simulink model "Simple_wanderer_local"  (R2013a)
settings: Solver=FixedStepDiscrete  StartTime=0.0  StopTime=300000  FixedStep=0.1  RelTol=1e-3
StopFcn:
  | arrobot_stop
libraries: ariac x8, simulink x1
PauseFcn:
  | arrobot_stop
settings Model: Creator=reedh  LastModifiedBy=reedh
settings DataIOCC: SaveFormat=StructureWithTime

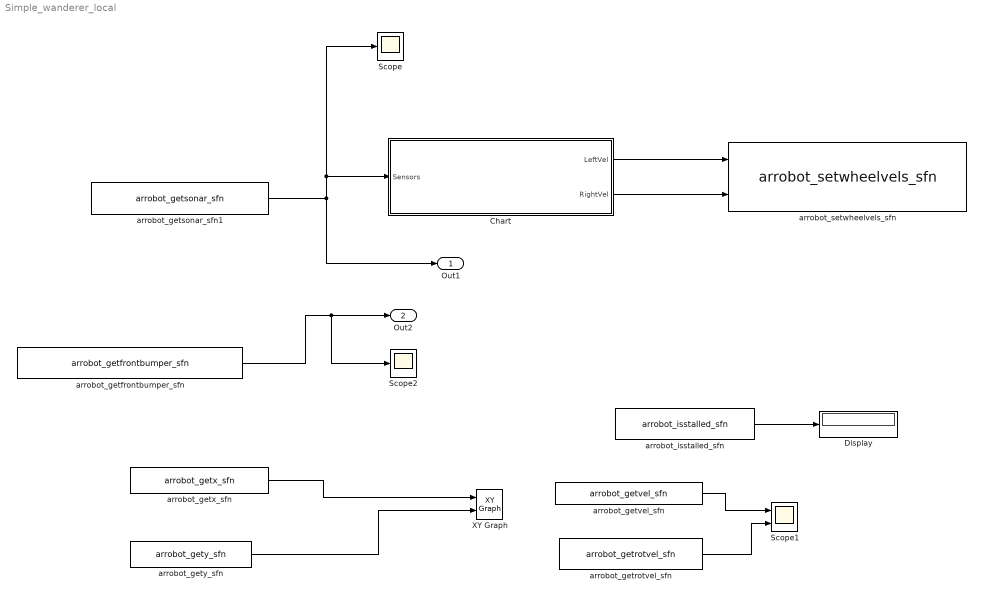
== system Simple_wanderer_local ==
  Chart : Stateflow chart  TreatAsAtomicUnit=on
  Display : Display
  Scope : Scope
      settings: YMin=0  YMax=5000
  Scope1 : Scope  NumInputPorts=2
      settings: YMin=-5~-5  YMax=5~5  SaveName=ScopeData2
  Scope2 : Scope
      settings: YMin=0  YMax=5000
  XY Graph : simulink/Sinks/XY Graph  xmin=-10000  xmax=10000  ymin=-10000  ymax=10000  st=100
  arrobot_getfrontbumper_sfn : ariac/arrobot_getfrontbumper_sfn  Description=Get range reading from one front bumper (0-indexed) of mobile robot  SFunctionSpec=int32 y1 = arrobot_get_front_bumper(int32 p1)  SParameter1=ones([1 1 ])  ShowSpec=on
      settings: AttributesFormatString=Get range reading from one front bumper (0-indexed) of mobile robot
  arrobot_getrotvel_sfn : ariac/arrobot_getrotvel_sfn  Description=Get current rotational velocity of mobile robot (deg/sec, counterclockwise +)  SFunctionSpec=double y1 = arrobot_getrotvel()  ShowSpec=on
      settings: AttributesFormatString=Get current rotational velocity of mobile robot (deg/sec, counterclockwise +)
  arrobot_getsonar_sfn1 : ariac/arrobot_getsonar_sfn  Description=Get range readings of all front sonar on mobile robot (mm)  SFunctionSpec=void arrobot_getsonar(double y1[16])  ShowSpec=on
      settings: AttributesFormatString=Get range readings of all front sonar on mobile robot (mm)
  arrobot_getvel_sfn : ariac/arrobot_getvel_sfn  Description=Get current forward/back velocity of mobile robot (mm/sec)  SFunctionSpec=double y1 = arrobot_getvel()  ShowSpec=on
      settings: AttributesFormatString=Get current forward/back velocity of mobile robot (mm/sec)
  arrobot_getx_sfn : ariac/arrobot_getx_sfn  Description=X position of mobile robot (mm)  SFunctionSpec=double y1 = arrobot_getx()  ShowSpec=on
      settings: AttributesFormatString=X position of mobile robot (mm)
  arrobot_gety_sfn : ariac/arrobot_gety_sfn  Description=Y position of mobile robot (mm)  SFunctionSpec=double y1 = arrobot_gety()  ShowSpec=on
      settings: AttributesFormatString=Y position of mobile robot (mm)
  arrobot_isstalled_sfn : ariac/arrobot_isstalled_sfn  Description=Are either motors stalled?  SFunctionSpec=int32 y1 = arrobot_isstalled()  ShowSpec=on
      settings: AttributesFormatString=Are either motors stalled?
  arrobot_setwheelvels_sfn : ariac/arrobot_setwheelvels_sfn  Description=Set left, right wheel velocities separately (mm/sec), overrides vel, rotvel  SFunctionSpec=void arrobot_setwheelvels(double u1, double u2)  ShowSpec=on
      settings: AttributesFormatString=Set left, right wheel velocities separately (mm/sec), overrides vel, rotvel
  Out1 : Outport
  Out2 : Outport  Port=2
  wires:
  Chart/1(LeftVel) -> arrobot_setwheelvels_sfn/1
  Chart/2(RightVel) -> arrobot_setwheelvels_sfn/2
  arrobot_getsonar_sfn1/1 -> Chart/1(Sensors), Scope/1, Out1/1
  arrobot_getfrontbumper_sfn/1 -> Scope2/1, Out2/1
  arrobot_getx_sfn/1 -> XY Graph/1
  arrobot_gety_sfn/1 -> XY Graph/2
  arrobot_getvel_sfn/1 -> Scope1/1
  arrobot_getrotvel_sfn/1 -> Scope1/2
  arrobot_isstalled_sfn/1 -> Display/1

== stateflow chart Simple_wanderer_local/Chart ==
  state Modes [parallel]
    en,du:
    v0 = 100;
    settings: executionOrder=1
    state GoStraight
      en, du:
      RightVel = v0;
      LeftVel = v0;
    state Turn
      en:
      num = 0;
      state TurnL
        en:
        num=num+1;
        du :
        RightVel = v0;
        LeftVel = -v0;
      state TurnR
        en:
        num=num+1;
        du :
        RightVel = -v0;
        LeftVel = v0;
      (default) -> TurnR
      TurnL -> TurnR [order 1] : RIGHT
      TurnR -> TurnL [order 1] : LEFT
      TurnL -> (junction 209) [order 2]
      TurnR -> (junction 209) [order 2]
      (junction 209) -> (junction 212) : [num > 3]{send(Modes.LOCK)}
    state GoStraight1
      en, du:
      RightVel = v0;
      LeftVel = v0;
    (default) -> GoStraight
    Turn -> GoStraight [order 1] : FORWARD
    GoStraight -> Turn : TURN
    Turn -> GoStraight1 [order 2] : LOCK
    GoStraight1 -> Turn : after(20,TURN)
  state ObjectDetection [parallel]
    en,du:
    settings: executionOrder=2
    state logic
      en,du:
      (default) -> (junction 2) : {   i=1;
          |     detect_st =0;
          |     detect_end=0;}
      (junction 2) -> (junction 45) [order 1] : [i < 8]
      (junction 45) -> (junction 11)
      (junction 11) -> (junction 10) [order 1] : [Sensors[i]<500]
      (junction 10) -> (junction 26)
      (junction 11) -> (junction 16) [order 2]
      (junction 26) -> (junction 27) [order 1] : [detect_st == 0]
      (junction 26) -> (junction 32) [order 2] : {detect_end = i;}
      (junction 27) -> (junction 33) : {detect_st=i;
          | detect_end=i;}
      (junction 40) -> (junction 2) : {i = i + 1;}
      (junction 2) -> (junction 5) [order 2]
      (junction 33) -> (junction 32)
      (junction 32) -> (junction 14)
      (junction 14) -> (junction 16)
      (junction 16) -> (junction 40)
      (junction 5) -> (junction 41) [order 1] : [detect_st !=0]
          | {send(Modes.TURN)}
      (junction 5) -> (junction 43) [order 2] : {send(Modes.FORWARD)}
      (junction 41) -> (junction 195)
      (junction 195) -> (junction 192) [order 1] : [detect_st < 4]
      (junction 195) -> (junction 190) [order 2] : {send(Modes.LEFT)}
      (junction 192) -> (junction 193) : {send(Modes.RIGHT)}
      (junction 193) -> (junction 190)
      (junction 190) -> (junction 197) : //{send(Modes.TURN)}
    (default) -> logic
    logic -> logic
  data: i local double size=1; LeftVel output; RightVel output; Sensors input size=16; v0 local double size=1; detect_st local double size=1; detect_end local double size=1; num local double
  events: FORWARD local FUNCTION_CALL_EVENT; RIGHT local FUNCTION_CALL_EVENT; LEFT local FUNCTION_CALL_EVENT; TURN local FUNCTION_CALL_EVENT; LOCK local FUNCTION_CALL_EVENT
